simulink model "Tiny_M28"  (R2017b)
settings: Solver=VariableStepAuto  StartTime=0.0  StopTime=10.0  RelTol=1e-3
settings Model: Creator=ainhoa.arruabarrena  LastModifiedBy=ainhoa.arruabarrena

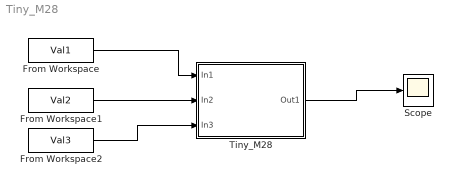
== system Tiny_M28 ==
  From Workspace : FromWorkspace  VariableName=Val1  SampleTime=0
  From Workspace1 : FromWorkspace  VariableName=Val2  SampleTime=0
  From Workspace2 : FromWorkspace  VariableName=Val3  SampleTime=0
  Scope : Scope
  Tiny_M28 : Subsystem
  wires:
  From Workspace2/1 -> Tiny_M28/3(In3)
  From Workspace1/1 -> Tiny_M28/2(In2)
  Tiny_M28/1(Out1) -> Scope/1
  From Workspace/1 -> Tiny_M28/1(In1)

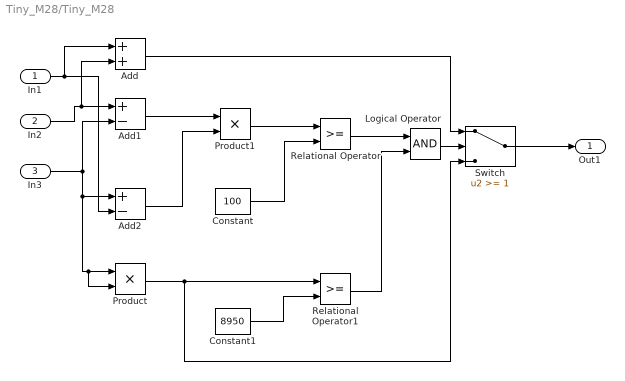
== system Tiny_M28/Tiny_M28 ==
  In1 : Inport
  In2 : Inport  Port=2
  In3 : Inport  Port=3
  Add : Sum
  Add1 : Sum  Inputs=+-
  Add2 : Sum  Inputs=+-
  Constant : Constant  Value=100
  Constant1 : Constant  Value=8950
  Logical Operator : Logic  AllPortsSameDT=off  OutDataTypeStr=boolean
  Product : Product
  Product1 : Product
  Relational Operator : RelationalOperator  OutDataTypeStr=boolean  RndMeth=Nearest
  Relational Operator1 : RelationalOperator  OutDataTypeStr=boolean  RndMeth=Nearest
  Switch : Switch  Threshold=1
  Out1 : Outport
  wires:
  Switch/1 -> Out1/1
  Add/1 -> Switch/1
  Logical Operator/1 -> Switch/2
  Relational Operator1/1 -> Logical Operator/2
  Relational Operator/1 -> Logical Operator/1
  Constant1/1 -> Relational Operator1/2
  Constant/1 -> Relational Operator/2
  Product/1 -> Relational Operator1/1, Switch/3
  Product1/1 -> Relational Operator/1
  Add2/1 -> Product1/2
  Add1/1 -> Product1/1
  In2/1 -> Add1/1, Add/2
  In1/1 -> Add2/2, Add/1
  In3/1 -> Add1/2, Product/1, Product/2, Add2/1
